simulink model "test1"  (R2020b)
settings: Solver=ode1  StartTime=0.0  StopTime=Inf  FixedStep=0.001  RelTol=1e-3
undefined symbols (not defined in the file or in its folder): kd, kd_best, ki, ki_best, kp, kp_best, mot, National_Instruments, PCIe, sens
libraries: sldrtlib x3, powerlib_meascontrol x1
settings Model: ExtModeTrigDuration=50000  Creator=pellizzar1  LastModifiedBy=pellizzar1
settings DataIOCC: ReturnWorkspaceOutputs=off
settings RTWCC: Description=Simulink Desktop Real-Time  SystemTargetFile=sldrt.tlc  TemplateMakefile=sldrt.tmf  RTWCompilerOptimization=on
settings CodeAppCC: MaxIdLength=95
settings SimulinkDesktopRealTimeCC: TargetPreCompLibLocation=C:\Program Files\MATLAB\R2020b\toolbox\sldrt\lib\win64

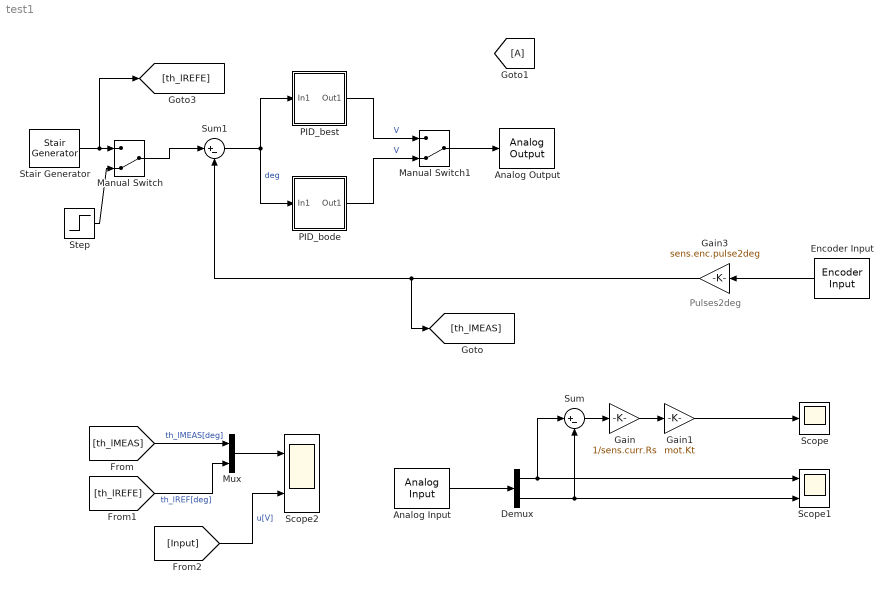
== system test1 ==
  note: Pulses2deg
  Analog Input : sldrtlib/Analog Input  SampleTime=0.001  MaxMissedTicks=10  ShowMissedTicks=off  YieldWhenWaiting=off  DrvName=National_Instruments/PCIe-6321  DrvAddress=4294967295  DrvOptions=[0 0 0 2 0 0 0]  Channels=[1,2]  RangeMode=1  VoltRange=1  DataType=1
      settings: AttributesFormatString=National Instruments\nPCIe-6321 [auto]
  Analog Output : sldrtlib/Analog Output  SampleTime=0.001  MaxMissedTicks=10  ShowMissedTicks=off  YieldWhenWaiting=off  DrvName=National_Instruments/PCIe-6321  DrvAddress=4294967295  DrvOptions=[0 0 0 2 0 0 0]  Channels=1  RangeMode=1  VoltRange=1  InitialValue=0  FinalValue=0
      settings: AttributesFormatString=National Instruments\nPCIe-6321 [auto]
  Demux : Demux  Outputs=2
  Encoder Input : sldrtlib/Encoder Input  SampleTime=0.001  MaxMissedTicks=10  ShowMissedTicks=off  YieldWhenWaiting=off  DrvName=National_Instruments/PCIe-6321  DrvAddress=4294967295  DrvOptions=[0 0 0 2 0 0 0]  Channels=1  QuadMode=3  IndexPulse=1  InputFilter=Inf  DataType=1
      settings: AttributesFormatString=National Instruments\nPCIe-6321 [auto]
  Gain : Gain  Gain=1/sens.curr.Rs
  Gain1 : Gain  Gain=mot.Kt
  Gain3 : Gain  Gain=sens.enc.pulse2deg
  Manual Switch : ManualSwitch  CurrentSetting=0
  Manual Switch1 : ManualSwitch  CurrentSetting=0
  Mux : Mux  Inputs=2
  PID_best : Subsystem
  PID_bode : Subsystem
  Scope : Scope
  Scope1 : Scope  NumInputPorts=2
  Scope2 : Scope  NumInputPorts=2
  Stair Generator : powerlib_meascontrol/Pulse & Signal Generators/Stair Generator  t=[0,2, 4, 6,8,10,12,14,16,18,20]  e=[10,0,30,0,50,0,90,0,180,0,360]  Ts=0
  Step : Step  Time=0  After=10  SampleTime=0
  Sum : Sum  Inputs=|+-
  Sum1 : Sum  Inputs=|+-
  wires:
  Analog Input/1 -> Demux/1
  Demux/1 -> Sum/1, Scope1/1
  Demux/2 -> Sum/2, Scope1/2
  Step/1 -> Manual Switch/2
  Manual Switch1/1 -> Analog Output/1
  Mux/1 -> Scope2/1
  [th_lREFE] -> Mux/2  "th_lREF[deg]"
  Manual Switch/1 -> Sum1/1
  PID_best/1(Out1) -> Manual Switch1/1  "V"
  [Input] -> Scope2/2  "u[V]"
  [th_lMEAS] -> Mux/1  "th_lMEAS[deg]"
  Gain3/1 -> Sum1/2, [th_lMEAS]
  Sum1/1 -> PID_best/1(In1), PID_bode/1(In1)  "deg"
  PID_bode/1(Out1) -> Manual Switch1/2  "V"
  Stair Generator/1 -> [th_lREFE], Manual Switch/1
  Encoder Input/1 -> Gain3/1
  Sum/1 -> Gain/1
  Gain/1 -> Gain1/1
  Gain1/1 -> Scope/1

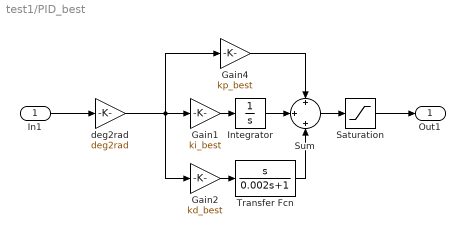
== system test1/PID_best ==
  In1 : Inport
  Gain1 : Gain  Gain=ki_best
  Gain2 : Gain  Gain=kd_best
  Gain4 : Gain  Gain=kp_best
  Integrator : Integrator
  Saturation : Saturate  UpperLimit=10  LowerLimit=-10
  Sum : Sum  Inputs=+|+|+
  Transfer Fcn : TransferFcn  Numerator=[1 0]  Denominator=[0.002 1]
  deg2rad : Gain  Gain=deg2rad
  Out1 : Outport
  wires:
  Transfer Fcn/1 -> Sum/3
  deg2rad/1 -> Gain1/1, Gain4/1, Gain2/1
  In1/1 -> deg2rad/1
  Gain2/1 -> Transfer Fcn/1
  Sum/1 -> Saturation/1
  Saturation/1 -> Out1/1
  Integrator/1 -> Sum/2
  Gain1/1 -> Integrator/1
  Gain4/1 -> Sum/1

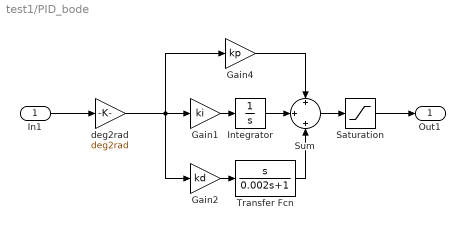
== system test1/PID_bode ==
  In1 : Inport
  Gain1 : Gain  Gain=ki
  Gain2 : Gain  Gain=kd
  Gain4 : Gain  Gain=kp
  Integrator : Integrator
  Saturation : Saturate  UpperLimit=10  LowerLimit=-10
  Sum : Sum  Inputs=+|+|+
  Transfer Fcn : TransferFcn  Numerator=[1 0]  Denominator=[0.002 1]
  deg2rad : Gain  Gain=deg2rad
  Out1 : Outport
  wires:
  Gain4/1 -> Sum/1
  Gain1/1 -> Integrator/1
  Integrator/1 -> Sum/2
  Saturation/1 -> Out1/1
  Sum/1 -> Saturation/1
  Gain2/1 -> Transfer Fcn/1
  In1/1 -> deg2rad/1
  deg2rad/1 -> Gain2/1, Gain4/1, Gain1/1
  Transfer Fcn/1 -> Sum/3
